simulink model "prob_4"  (R2020b)
settings: Solver=VariableStepAuto  StartTime=0.0  StopTime=10.0  RelTol=1e-3
settings Model: Creator=Akshay A H  LastModifiedBy=Akshay A H

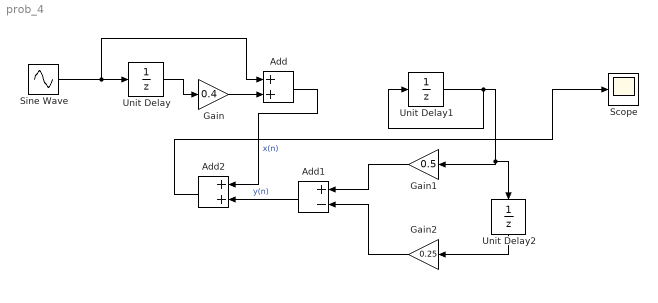
== system prob_4 ==
  Add : Sum
  Add1 : Sum  Inputs=+-
  Add2 : Sum
  Gain : Gain  Gain=0.4
  Gain1 : Gain  Gain=0.5
  Gain2 : Gain  Gain=0.25
  Scope : Scope
  Sine Wave : Sin  SampleTime=0
  Unit Delay : UnitDelay  SampleTime=-1  HasFrameUpgradeWarning=on
  Unit Delay1 : UnitDelay  SampleTime=-1  HasFrameUpgradeWarning=on
  Unit Delay2 : UnitDelay  SampleTime=-1  HasFrameUpgradeWarning=on
  wires:
  Sine Wave/1 -> Unit Delay/1, Add/1
  Unit Delay/1 -> Gain/1
  Gain/1 -> Add/2
  Unit Delay1/1 -> Unit Delay1/1, Unit Delay2/1, Gain1/1
  Unit Delay2/1 -> Gain2/1
  Gain2/1 -> Add1/2
  Gain1/1 -> Add1/1
  Add/1 -> Add2/1  "x(n)"
  Add1/1 -> Add2/2  "y(n)"
  Add2/1 -> Scope/1
